simulink model "state_reg_mdl_2023a"  (R2023a)
settings: Solver=VariableStepAuto  StartTime=0.0  StopTime=20  RelTol=1e-3
StartFcn:
  | state_reg
values from neighbouring files (symbols this model uses):
  K = acker(A, B, p)    [state_reg.m]
  T = 1e-3    (= 0.001)    [state_reg.m]
  umax = 1    [state_reg.m]
libraries: simulink x1
settings Model: Creator=rapaja  LastModifiedBy=Predrag
settings SolverCC: AlgebraicLoopSolver=TrustRegion
settings DebuggingCC: UnconnectedInputMsg=warning  UnconnectedOutputMsg=warning  UnconnectedLineMsg=warning
settings ModelReferenceCC: EnableRefExpFcnMdlSchedulingChecks=on
settings ConfigComp: CovBoundaryAbsTol=1.0e-5

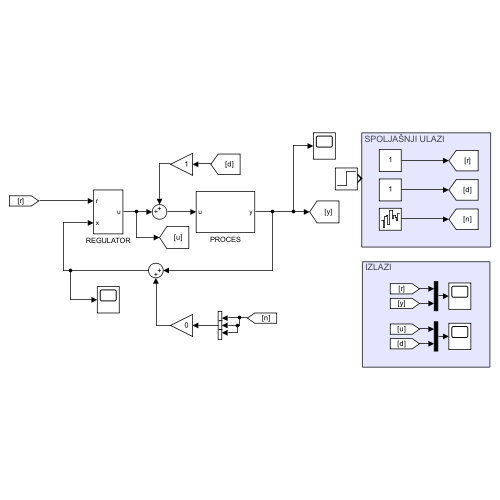
[thumbnail: Simulink's stored preview of the top-level diagram]
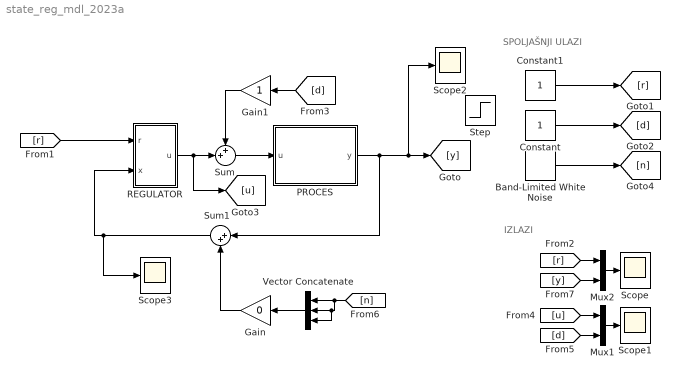
== system state_reg_mdl_2023a ==
  note: IZLAZI
  note: SPOLJAŠNJI ULAZI
  Band-Limited White Noise : simulink/Sources/Band-Limited White Noise  Cov=[0.00001]  Ts=T  seed=[23341]
  Constant : Constant
  Constant1 : Constant
  Gain : Gain  Gain=0
  Gain1 : Gain
  Mux1 : Mux  Inputs=2
  Mux2 : Mux  Inputs=2
  PROCES : Subsystem
  REGULATOR : Subsystem
  Scope{,1..3} (4 alike) : Scope
  Step : Step  After=0  SampleTime=0
  Sum : Sum  Inputs=++|
  Sum1 : Sum  Inputs=|++
  Vector Concatenate : Concatenate  NumInputs=3
  wires:
  REGULATOR/1(u) -> Sum/2, [u]
  [d] -> Gain1/1
  Band-Limited White Noise/1 -> [n]
  Gain/1 -> Sum1/2
  Gain1/1 -> Sum/1
  Constant/1 -> [d]
  [r] -> Mux2/1
  [y] -> Mux2/2
  Mux2/1 -> Scope/1
  Mux1/1 -> Scope1/1
  [u] -> Mux1/1
  [d] -> Mux1/2
  PROCES/1(y) -> Sum1/1, Scope2/1, [y]
  [r] -> REGULATOR/1(r)
  Sum/1 -> PROCES/1(u)
  Sum1/1 -> Scope3/1, REGULATOR/2(x)
  [n] -> Vector Concatenate/3, Vector Concatenate/2, Vector Concatenate/1
  Vector Concatenate/1 -> Gain/1
  Constant1/1 -> [r]

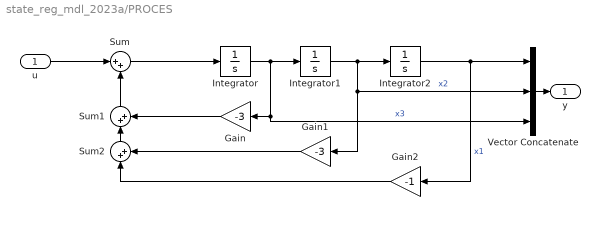
== system state_reg_mdl_2023a/PROCES ==
  u : Inport
  Gain : Gain  Gain=-3
  Gain1 : Gain  Gain=-3
  Gain2 : Gain  Gain=-1
  Integrator : Integrator
  Integrator1 : Integrator
  Integrator2 : Integrator
  Sum : Sum  Inputs=|++
  Sum1 : Sum  Inputs=|++
  Sum2 : Sum  Inputs=|++
  Vector Concatenate : Concatenate  NumInputs=3
  y : Outport
  wires:
  Vector Concatenate/1 -> y/1
  Integrator2/1 -> Gain2/1, Vector Concatenate/1  "x1"
  Integrator1/1 -> Vector Concatenate/2, Gain1/1, Integrator2/1  "x2"
  Integrator/1 -> Vector Concatenate/3, Gain/1, Integrator1/1  "x3"
  u/1 -> Sum/1
  Sum/1 -> Integrator/1
  Gain/1 -> Sum1/2
  Sum1/1 -> Sum/2
  Sum2/1 -> Sum1/1
  Gain1/1 -> Sum2/2
  Gain2/1 -> Sum2/1

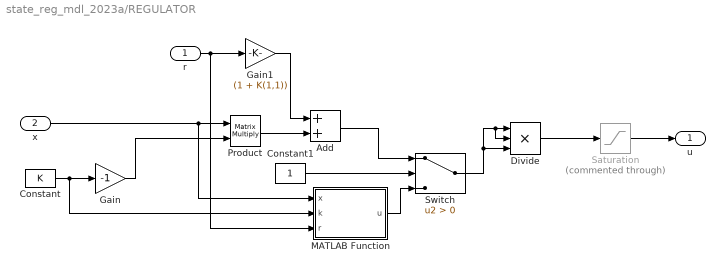
== system state_reg_mdl_2023a/REGULATOR ==
  r : Inport
  x : Inport  Port=2
  Add : Sum
  Constant : Constant  Value=K
  Constant1 : Constant
  Divide : Product  Inputs=***
  Gain : Gain  Gain=-1
  Gain1 : Gain  Gain=(1 + K(1,1))
  MATLAB Function : MATLAB Function  TreatAsAtomicUnit=on  SystemSampleTime=T
  Product : Product  Multiplication=Matrix(*)
  Saturation : Saturate  Commented=through  UpperLimit=umax  LowerLimit=-umax
  Switch : Switch  Criteria=u2 > Threshold  SaturateOnIntegerOverflow=off  InputSameDT=off
  u : Outport
  wires:
  Saturation/1 -> u/1
  Constant/1 -> MATLAB Function/2(k), Gain/1
  r/1 -> Gain1/1, MATLAB Function/3(r)
  Gain1/1 -> Add/1
  Product/1 -> Add/2
  Gain/1 -> Product/2
  x/1 -> MATLAB Function/1(x), Product/1
  Divide/1 -> Saturation/1
  Switch/1 -> Divide/3, Divide/2, Divide/1
  MATLAB Function/1(u) -> Switch/3
  Add/1 -> Switch/1
  Constant1/1 -> Switch/2

== matlab function state_reg_mdl_2023a/REGULATOR/MATLAB Function ==
  data: x input; u output; k input; r input
function u = fcn(x, k, r)

u = -transpose(k)*x + 1/(1 + k(1, 1)) * r;
